simulink model "FOC_Motor_Control"  (R2020b)
settings: Solver=FixedStepAuto  StartTime=0.0  StopTime=10.0  FixedStep=Fixed_Step_Size  RelTol=1e-3
values from neighbouring files (symbols this model uses):
  atan_table = -1.5690511 -1.5690503 -1.5690495 -1.5690485 -1.5690477 -1.5690469 -1.569046 -1.5690452 -1.5690442 -1.5690434 -1.5690426 -1.5690417 -1.5690409 -1.5690399 -1.5690391 -1.5690383 -1.5690374 -1.5690365 -1.5690356 -1.5690348 -1.5690339 -1.569033 -1.5690322 -1.5690314 -1.5690304 -1.5690296 -1.5690287 -1.5690278 -1.5690269 -1.5690261 -1.5690252 -1.5690243 -1.5690234 -1.5690225 -1.5690217 -1.5690207 -1.569    [Motor_Control_Data.sldd]
  Cosine_table = 1.0 0.99999529 0.99999058 0.99998587 0.99998116 0.99996704 0.99995291 0.99993885 0.99992472 0.99990118 0.99987763 0.99985409 0.9998306 0.99979764 0.99976468 0.99973178 0.99969882 0.99965644 0.99961412 0.99957174 0.99952942 0.99947762 0.99942589 0.99937415 0.99932235 0.9992612 0.99920005 0.99913889 0.99907768 0.99900717 0.99893659 0.99886602 0.99879545 0.99871546 0.99863547 0.99855554 0.99847555 0.    [Motor_Control_Data.sldd]
  Dead_Com_Enable = 1.0    [Motor_Control_Data.sldd]
  Dead_Time = 2.5E-6    [Motor_Control_Data.sldd]
  Flux = 0.1125    [Motor_Control_Data.sldd]
  ID_Ki = 48.0    [Motor_Control_Data.sldd]
  ID_Kp = 0.84    [Motor_Control_Data.sldd]
  IQ_Ki = 48.0    [Motor_Control_Data.sldd]
  IQ_Kp = 1.869    [Motor_Control_Data.sldd]
  Ld = 0.00014    [Motor_Control_Data.sldd]
  Lq = 0.0003115    [Motor_Control_Data.sldd]
  Pole_Pairs = 4.0    [Motor_Control_Data.sldd]
  PWM_Frequency = 10000.0    [Motor_Control_Data.sldd]
  Sine_table = 0.0 0.0015339879 0.0030679768 0.0046019657 0.0061359555 0.0076698866 0.0092038177 0.010737749 0.012271681 0.013805497 0.015339312 0.016873131 0.018406944 0.019940587 0.021474229 0.023007872 0.024541514 0.026074925 0.027608337 0.029141748 0.03067516 0.032208283 0.033741407 0.035274528 0.036807653 0.038340431 0.039873205 0.04140598 0.042938754 0.04447113 0.046003502 0.047535874 0.049068246 0.0506001    [Motor_Control_Data.sldd]
  Speed_Ki = 10.809    [Motor_Control_Data.sldd]
  Speed_Kp = 0.08    [Motor_Control_Data.sldd]
  Speed_PI_OutputMax = 700.0    [Motor_Control_Data.sldd]
  Speed_PI_OutputMin = -700.0    [Motor_Control_Data.sldd]
  SpeedFilter_Fn = 0.2    [Motor_Control_Data.sldd]
  TorqueMode = 0.0    [Motor_Control_Data.sldd]
undefined symbols (not defined in the file or in its folder): DiscIntNeverNeededParam, inverter, LADRC_b0, LADRC_Omega_c, SVPWM
libraries: simulink x6
(part 2 of 2)

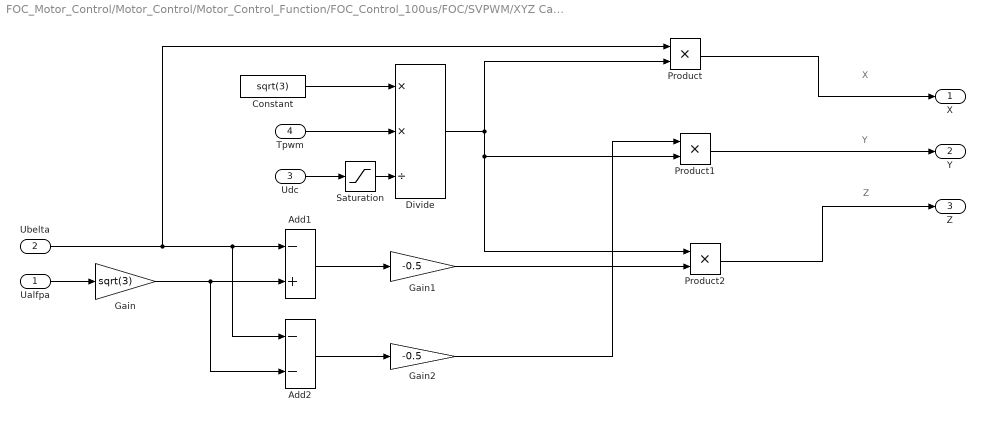
== system FOC_Motor_Control/Motor_Control/Motor_Control_Function/FOC_Control_100us/FOC/SVPWM/XYZ Caculate ==
  note: X
  note: Y
  note: Z
  Ualfpa : Inport
  Ubelta : Inport  Port=2
  Udc : Inport  Port=3
  Tpwm : Inport  Port=4
  Add1 : Sum  Inputs=-+
  Add2 : Sum  Inputs=--
  Constant : Constant  Value=sqrt(3)  OutDataTypeStr=single
  Divide : Product  Inputs=**/
  Gain : Gain  Gain=sqrt(3)
  Gain1 : Gain  Gain=-0.5
  Gain2 : Gain  Gain=-0.5
  Product : Product
  Product1 : Product
  Product2 : Product
  Saturation : Saturate  UpperLimit=1200  LowerLimit=0.0001
  X : Outport
  Y : Outport  Port=2
  Z : Outport  Port=3
  wires:
  Gain2/1 -> Product1/1
  Add2/1 -> Gain2/1
  Add1/1 -> Gain1/1
  Gain/1 -> Add2/2, Add1/2
  Ualfpa/1 -> Gain/1
  Ubelta/1 -> Add2/1, Add1/1, Product/1
  Gain1/1 -> Product2/2
  Product2/1 -> Z/1
  Divide/1 -> Product1/2, Product2/1, Product/2
  Product1/1 -> Y/1
  Product/1 -> X/1
  Udc/1 -> Saturation/1
  Tpwm/1 -> Divide/2
  Constant/1 -> Divide/1
  Saturation/1 -> Divide/3

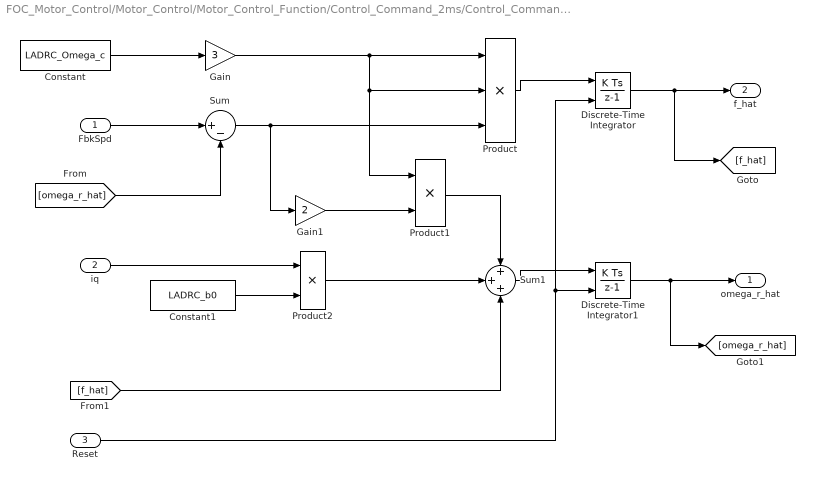
== system FOC_Motor_Control/Motor_Control/Motor_Control_Function/Control_Command_2ms/Control_Command_2ms/Speed_PI/SpeedLoop/LESO ==
  FbkSpd : Inport  OutDataTypeStr=single  PortDimensions=1
  iq : Inport  Port=2  OutDataTypeStr=single  PortDimensions=1
  Reset : Inport  Port=3
  Constant : Constant  Value=LADRC_Omega_c  OutDataTypeStr=single
  Constant1 : Constant  Value=LADRC_b0  OutDataTypeStr=single  SampleTime=-1
  Discrete-Time Integrator : DiscreteIntegrator  ExternalReset=level  SampleTime=-1  OutDataTypeStr=single  UpperSaturationLimit=6e4  LowerSaturationLimit=-6e4  ICPrevOutput=DiscIntNeverNeededParam  ICPrevScaledInput=DiscIntNeverNeededParam
  Discrete-Time Integrator1 : DiscreteIntegrator  ExternalReset=level  SampleTime=-1  OutDataTypeStr=single  LimitOutput=on  UpperSaturationLimit=2000  LowerSaturationLimit=-2000  ICPrevOutput=DiscIntNeverNeededParam  ICPrevScaledInput=DiscIntNeverNeededParam
  Gain : Gain  Gain=3  OutDataTypeStr=single
  Gain1 : Gain  Gain=2  OutDataTypeStr=single
  Product : Product  Inputs=3  OutDataTypeStr=single
  Product1 : Product  OutDataTypeStr=single
  Product2 : Product  OutDataTypeStr=single
  Sum : Sum  Inputs=|+-  OutDataTypeStr=single
  Sum1 : Sum  Inputs=+++  OutDataTypeStr=single
  omega_r_hat : Outport  OutDataTypeStr=single
  f_hat : Outport  Port=2  OutDataTypeStr=single
  wires:
  Sum/1 -> Gain1/1, Product/3
  Product/1 -> Discrete-Time Integrator/1
  Discrete-Time Integrator/1 -> [f_hat], f_hat/1
  [f_hat] -> Sum1/3
  Sum1/1 -> Discrete-Time Integrator1/1
  Discrete-Time Integrator1/1 -> omega_r_hat/1, [omega_r_hat]
  Product1/1 -> Sum1/1
  FbkSpd/1 -> Sum/1
  [omega_r_hat] -> Sum/2
  Constant/1 -> Gain/1
  Gain1/1 -> Product1/2
  Gain/1 -> Product1/1, Product/2, Product/1
  iq/1 -> Product2/1
  Constant1/1 -> Product2/2
  Product2/1 -> Sum1/2
  Reset/1 -> Discrete-Time Integrator/2, Discrete-Time Integrator1/2

== system FOC_Motor_Control/Motor_Control/Motor_Control_Function/Control_Command_2ms/Control_Command_2ms/Speed_PI/Speed_PI/Speed_Control ==
  Err : Inport
  Reset : Inport  Port=2
  Add : Sum
  Cons : Constant  Value=0  OutDataTypeStr=single
  Discrete-Time Integrator : DiscreteIntegrator  ExternalReset=level  SampleTime=-1  ICPrevOutput=DiscIntNeverNeededParam  ICPrevScaledInput=DiscIntNeverNeededParam
  Ki : Constant  Value=Speed_Ki  OutDataTypeStr=single
  Kp : Constant  Value=Speed_Kp  OutDataTypeStr=single
  Product : Product
  Product1 : Product
  Relational Operator1 : RelationalOperator  Operator===  OutDataTypeStr=boolean  RndMeth=Simplest
  Saturation : Saturate  UpperLimit=Speed_PI_OutputMax  LowerLimit=Speed_PI_OutputMin
  Scope : Scope
  Switch : Switch  Criteria=u2 > Threshold
  Unit Delay3 : UnitDelay  SampleTime=-1  HasFrameUpgradeWarning=on
  PI_Out : Outport
  wires:
  Kp/1 -> Product/1
  Err/1 -> Switch/1, Product/2
  Switch/1 -> Product1/2
  Product1/1 -> Discrete-Time Integrator/1
  Product/1 -> Add/1
  Add/1 -> Relational Operator1/1, Saturation/1
  Saturation/1 -> Relational Operator1/2, PI_Out/1
  Discrete-Time Integrator/1 -> Add/2, Scope/1
  Relational Operator1/1 -> Unit Delay3/1
  Ki/1 -> Product1/1
  Unit Delay3/1 -> Switch/2
  Cons/1 -> Switch/3
  Reset/1 -> Discrete-Time Integrator/2

== system FOC_Motor_Control/Motor_Control/Motor_Control_Function/FOC_Control_100us/FOC/DT_Compensation/DT_Compensation/IsTheta_Cal ==
  Id : Inport
  Iq : Inport  Port=2
  d_theta : Inport  Port=3
  Add1 : Sum
  Angle_calibration : Subsystem
      settings: RTWSystemCode=Nonreusable function  RTWFcnNameOpts=Use subsystem name
  LPF : Subsystem
  LPF1 : Subsystem
  Scope2 : Scope  NumInputPorts=2
  Scope3 : Scope  NumInputPorts=2
  atan : Subsystem
  IsTheta : Outport
  wires:
  d_theta/1 -> Add1/2
  Angle_calibration/1(Angle_output) -> IsTheta/1
  Iq/1 -> LPF/1(u), Scope2/1
  Id/1 -> LPF1/1(u), Scope3/1
  LPF1/1(y) -> [B_Id], Scope3/2
  LPF/1(y) -> Scope2/2, [A_Iq]
  Add1/1 -> Angle_calibration/1(Angle_input)  "Itheta2"
  [A_Iq] -> atan/1(Id)
  [B_Id] -> atan/2(Iq)
  atan/1(Out1) -> Add1/1

== system FOC_Motor_Control/Motor_Control/Motor_Control_Function/FOC_Control_100us/FOC/DT_Compensation/DT_Compensation/Subsystem ==
  Err_Voltage : Inport
  Istheta : Inport  Port=2
  If1 : If  IfExpression=(u1 >5.75958)|(u1<=0.523598)  ElseIfExpressions=(u1 >0.523598)&(u1<=1.570796),(u1 >1.570796)&(u1<=2.617993),(u1 >2.617993)&(u1<=3.665191),(u1 >3.665191)&(u1<=4.7123889),(u1 >4.7123889)&(u1<=5.75958)  ShowElse=off
  Merge : Merge  Inputs=6
  Subsystem : Subsystem
  Subsystem1 : Subsystem
  Subsystem2 : Subsystem
  Subsystem3 : Subsystem
  Subsystem4 : Subsystem
  Subsystem5 : Subsystem
  Uabcc : Outport
  wires:
  Istheta/1 -> If1/1
  If1/1 -> Subsystem/Action
  If1/2 -> Subsystem1/Action
  If1/3 -> Subsystem2/Action
  If1/4 -> Subsystem3/Action
  If1/5 -> Subsystem4/Action
  If1/6 -> Subsystem5/Action
  Err_Voltage/1 -> Subsystem5/1(Voltage), Subsystem3/1(Voltage), Subsystem2/1(Voltage), Subsystem/1(Voltage), Subsystem1/1(Voltage), Subsystem4/1(Voltage)
  Merge/1 -> Uabcc/1
  Subsystem/1(Out1) -> Merge/1
  Subsystem1/1(Out1) -> Merge/2
  Subsystem2/1(Out1) -> Merge/3
  Subsystem3/1(Out1) -> Merge/4
  Subsystem4/1(Out1) -> Merge/5
  Subsystem5/1(Out1) -> Merge/6

== system FOC_Motor_Control/Motor_Control/Motor_Control_Function/FOC_Control_100us/FOC/DT_Compensation/DT_Compensation/Uabc_alphabeta ==
  Uabc : Inport
  Fcn : Fcn  Expr=(2/3)*(u(1)-0.5*u(2)-0.5*u(3))
  Fcn1 : Fcn  Expr=sqrt(1/3)*(u(2)-u(3))
  Ualpha : Outport
  Ubeta : Outport  Port=2
  wires:
  Fcn/1 -> Ualpha/1
  Fcn1/1 -> Ubeta/1
  Uabc/1 -> Fcn1/1, Fcn/1

== system FOC_Motor_Control/Motor_Control/Motor_Control_Function/FOC_Control_100us/FOC/D_Current_PI/ID_Control/Normal ==
  Bus_voltage : Inport
  Gain : Gain  Gain=1/sqrt(3)
  Gain1 : Gain  Gain=-1/sqrt(3)
  Out1 : Outport
  Out2 : Outport  Port=2
  wires:
  Bus_voltage/1 -> Gain1/1, Gain/1
  Gain/1 -> Out1/1
  Gain1/1 -> Out2/1

== system FOC_Motor_Control/Motor_Control/Motor_Control_Function/FOC_Control_100us/FOC/Q_Current_PI/IQ_Control/Normal ==
  Bus_voltage : Inport
  Gain : Gain  Gain=1/sqrt(3)
  Gain1 : Gain  Gain=-1/sqrt(3)
  Out1 : Outport
  Out2 : Outport  Port=2
  wires:
  Bus_voltage/1 -> Gain1/1, Gain/1
  Gain/1 -> Out1/1
  Gain1/1 -> Out2/1

== system FOC_Motor_Control/Motor_Control/Motor_Control_Function/FOC_Control_100us/FOC/DT_Compensation/DT_Compensation/IsTheta_Cal/Angle_calibration ==
  Angle_input : Inport
  If Action Subsystem1 : Subsystem  TreatAsAtomicUnit=on
  If Action Subsystem2 : Subsystem  TreatAsAtomicUnit=on
  If1 : If  IfExpression=u1 > 6.283185307
  Merge1 : Merge
  Angle_output : Outport
  wires:
  Merge1/1 -> Angle_output/1
  If1/1 -> If Action Subsystem2/Action
  If1/2 -> If Action Subsystem1/Action
  If Action Subsystem2/1(Out1) -> Merge1/1
  Angle_input/1 -> If Action Subsystem1/1(Angle_input), If Action Subsystem2/1(In1), If1/1
  If Action Subsystem1/1(Out1) -> Merge1/2

== system FOC_Motor_Control/Motor_Control/Motor_Control_Function/FOC_Control_100us/FOC/DT_Compensation/DT_Compensation/IsTheta_Cal/LPF ==
  u : Inport
  Add : Sum  Inputs=+-
  Add1 : Sum
  Constant1 : Constant  Value=0.005  OutDataTypeStr=single
  Divide1 : Product  Inputs=**
  Unit Delay : UnitDelay  SampleTime=-1  HasFrameUpgradeWarning=on
  y : Outport
  wires:
  Constant1/1 -> Divide1/1
  u/1 -> Add/1
  Add/1 -> Divide1/2
  Divide1/1 -> Add1/1
  Unit Delay/1 -> Add/2, Add1/2
  Add1/1 -> Unit Delay/1, y/1

== system FOC_Motor_Control/Motor_Control/Motor_Control_Function/FOC_Control_100us/FOC/DT_Compensation/DT_Compensation/IsTheta_Cal/LPF1 ==
  u : Inport
  Add : Sum  Inputs=+-
  Add1 : Sum
  Constant1 : Constant  Value=0.005  OutDataTypeStr=single
  Divide1 : Product  Inputs=**
  Unit Delay : UnitDelay  SampleTime=-1  HasFrameUpgradeWarning=on
  y : Outport
  wires:
  Constant1/1 -> Divide1/1
  u/1 -> Add/1
  Add/1 -> Divide1/2
  Divide1/1 -> Add1/1
  Unit Delay/1 -> Add/2, Add1/2
  Add1/1 -> Unit Delay/1, y/1

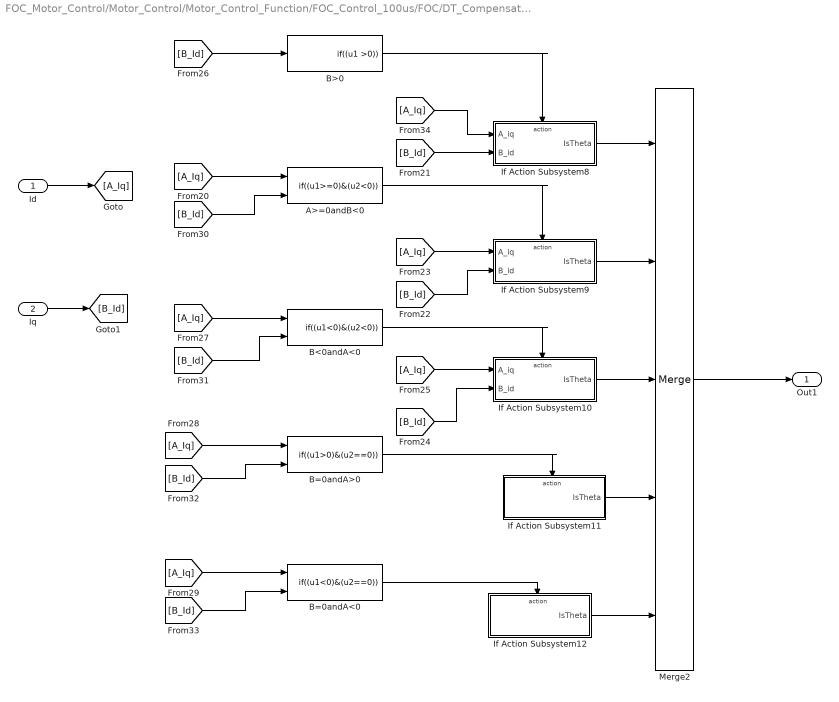
== system FOC_Motor_Control/Motor_Control/Motor_Control_Function/FOC_Control_100us/FOC/DT_Compensation/DT_Compensation/IsTheta_Cal/atan ==
  Id : Inport
  Iq : Inport  Port=2
  A>=0andB<0 : If  NumInputs=2  IfExpression=(u1>=0)&(u2<0)  ShowElse=off
  B<0andA<0 : If  NumInputs=2  IfExpression=(u1<0)&(u2<0)  ShowElse=off
  B=0andA<0 : If  NumInputs=2  IfExpression=(u1<0)&(u2==0)  ShowElse=off
  B=0andA>0 : If  NumInputs=2  IfExpression=(u1>0)&(u2==0)  ShowElse=off
  B>0 : If  IfExpression=(u1 >0)  ShowElse=off
  If Action Subsystem10 : Subsystem  TreatAsAtomicUnit=on
  If Action Subsystem11 : Subsystem  TreatAsAtomicUnit=on
  If Action Subsystem12 : Subsystem  TreatAsAtomicUnit=on
  If Action Subsystem8 : Subsystem  TreatAsAtomicUnit=on
  If Action Subsystem9 : Subsystem  TreatAsAtomicUnit=on
  Merge2 : Merge  Inputs=5
  Out1 : Outport
  wires:
  B<0andA<0/1 -> If Action Subsystem10/Action
  [A_Iq] -> If Action Subsystem10/1(A_iq)
  B=0andA<0/1 -> If Action Subsystem12/Action
  B=0andA>0/1 -> If Action Subsystem11/Action
  [A_Iq] -> If Action Subsystem8/1(A_iq)
  [B_Id] -> B>0/1
  A>=0andB<0/1 -> If Action Subsystem9/Action
  If Action Subsystem11/1(IsTheta) -> Merge2/4
  If Action Subsystem9/1(IsTheta) -> Merge2/2
  [B_Id] -> If Action Subsystem9/2(B_id)
  B>0/1 -> If Action Subsystem8/Action
  [A_Iq] -> If Action Subsystem9/1(A_iq)
  If Action Subsystem8/1(IsTheta) -> Merge2/1
  [B_Id] -> B<0andA<0/2
  [A_Iq] -> A>=0andB<0/1
  [B_Id] -> B=0andA<0/2
  [B_Id] -> A>=0andB<0/2
  [A_Iq] -> B=0andA<0/1
  [A_Iq] -> B=0andA>0/1
  [A_Iq] -> B<0andA<0/1
  [B_Id] -> B=0andA>0/2
  If Action Subsystem12/1(IsTheta) -> Merge2/5
  If Action Subsystem10/1(IsTheta) -> Merge2/3
  Merge2/1 -> Out1/1
  [B_Id] -> If Action Subsystem8/2(B_id)
  [B_Id] -> If Action Subsystem10/2(B_id)
  Id/1 -> [A_Iq]
  Iq/1 -> [B_Id]

== system FOC_Motor_Control/Motor_Control/Motor_Control_Function/FOC_Control_100us/FOC/DT_Compensation/DT_Compensation/Subsystem/Subsystem ==
  Voltage : Inport
  Action Port : ActionPort  ActionPortLabel=if((u1 >5.75958)|(u1<=0.523598))
  Gain : Gain
  Gain1 : Gain  Gain=-1
  Gain2 : Gain  Gain=-1
  Mux1 : Mux  Inputs=3
  Out1 : Outport
  wires:
  Gain/1 -> Mux1/1
  Gain1/1 -> Mux1/2
  Voltage/1 -> Gain2/1, Gain1/1, Gain/1
  Gain2/1 -> Mux1/3
  Mux1/1 -> Out1/1

== system FOC_Motor_Control/Motor_Control/Motor_Control_Function/FOC_Control_100us/FOC/DT_Compensation/DT_Compensation/Subsystem/Subsystem1 ==
  Voltage : Inport
  Action Port : ActionPort  ActionPortLabel=elseif((u1 >0.523598)&(u1<=1.570796))
  Gain : Gain
  Gain1 : Gain
  Gain2 : Gain  Gain=-1
  Mux1 : Mux  Inputs=3
  Out1 : Outport
  wires:
  Mux1/1 -> Out1/1
  Voltage/1 -> Gain2/1, Gain1/1, Gain/1
  Gain/1 -> Mux1/1
  Gain1/1 -> Mux1/2
  Gain2/1 -> Mux1/3

== system FOC_Motor_Control/Motor_Control/Motor_Control_Function/FOC_Control_100us/FOC/DT_Compensation/DT_Compensation/Subsystem/Subsystem2 ==
  Voltage : Inport
  Action Port : ActionPort  ActionPortLabel=elseif((u1 >1.570796)&(u1<=2.617993))
  Gain : Gain  Gain=-1
  Gain1 : Gain
  Gain2 : Gain  Gain=-1
  Mux1 : Mux  Inputs=3
  Out1 : Outport
  wires:
  Mux1/1 -> Out1/1
  Voltage/1 -> Gain2/1, Gain1/1, Gain/1
  Gain/1 -> Mux1/1
  Gain1/1 -> Mux1/2
  Gain2/1 -> Mux1/3

== system FOC_Motor_Control/Motor_Control/Motor_Control_Function/FOC_Control_100us/FOC/DT_Compensation/DT_Compensation/Subsystem/Subsystem3 ==
  Voltage : Inport
  Action Port : ActionPort  ActionPortLabel=elseif((u1 >2.617993)&(u1<=3.665191))
  Gain : Gain  Gain=-1
  Gain1 : Gain
  Gain2 : Gain
  Mux1 : Mux  Inputs=3
  Out1 : Outport
  wires:
  Mux1/1 -> Out1/1
  Voltage/1 -> Gain2/1, Gain1/1, Gain/1
  Gain/1 -> Mux1/1
  Gain1/1 -> Mux1/2
  Gain2/1 -> Mux1/3

== system FOC_Motor_Control/Motor_Control/Motor_Control_Function/FOC_Control_100us/FOC/DT_Compensation/DT_Compensation/Subsystem/Subsystem4 ==
  Voltage : Inport
  Action Port : ActionPort  ActionPortLabel=elseif((u1 >3.665191)&(u1<=4.7123889))
  Gain : Gain  Gain=-1
  Gain1 : Gain  Gain=-1
  Gain2 : Gain
  Mux1 : Mux  Inputs=3
  Out1 : Outport
  wires:
  Mux1/1 -> Out1/1
  Voltage/1 -> Gain2/1, Gain1/1, Gain/1
  Gain/1 -> Mux1/1
  Gain1/1 -> Mux1/2
  Gain2/1 -> Mux1/3

== system FOC_Motor_Control/Motor_Control/Motor_Control_Function/FOC_Control_100us/FOC/DT_Compensation/DT_Compensation/Subsystem/Subsystem5 ==
  Voltage : Inport
  Action Port : ActionPort  ActionPortLabel=elseif((u1 >4.7123889)&(u1<=5.75958))
  Gain : Gain
  Gain1 : Gain  Gain=-1
  Gain2 : Gain
  Mux1 : Mux  Inputs=3
  Out1 : Outport
  wires:
  Mux1/1 -> Out1/1
  Voltage/1 -> Gain2/1, Gain1/1, Gain/1
  Gain/1 -> Mux1/1
  Gain1/1 -> Mux1/2
  Gain2/1 -> Mux1/3

== system FOC_Motor_Control/Motor_Control/Motor_Control_Function/FOC_Control_100us/FOC/DT_Compensation/DT_Compensation/IsTheta_Cal/Angle_calibration/If Action Subsystem1 ==
  Angle_input : Inport
  Action Port : ActionPort  ActionPortLabel=else
  Out1 : Outport
  wires:
  Angle_input/1 -> Out1/1

== system FOC_Motor_Control/Motor_Control/Motor_Control_Function/FOC_Control_100us/FOC/DT_Compensation/DT_Compensation/IsTheta_Cal/Angle_calibration/If Action Subsystem2 ==
  In1 : Inport
  Action Port : ActionPort  ActionPortLabel=if(u1 > 6.283185307)
  2pi : Constant  Value=2*pi  OutDataTypeStr=single
  Subtract1 : Sum  Inputs=+-
  Out1 : Outport
  wires:
  In1/1 -> Subtract1/1
  Subtract1/1 -> Out1/1
  2pi/1 -> Subtract1/2

== system FOC_Motor_Control/Motor_Control/Motor_Control_Function/FOC_Control_100us/FOC/DT_Compensation/DT_Compensation/IsTheta_Cal/atan/If Action Subsystem10 ==
  A_iq : Inport
  B_id : Inport  Port=2
  Action Port : ActionPort  ActionPortLabel=if((u1<0)&(u2<0))
  1-D Lookup Table4 : Lookup_n-D  NumberOfTableDimensions=1  LookupTableObject=''  BreakpointsForDimension1=single(linspace(-573,573,length(atan_table)));  BreakpointsForDimension1FirstPoint=10  BreakpointsForDimension2FirstPoint=10  BreakpointsForDimension1Spacing=12  BreakpointsForDimension2Spacing=12  IndexSearchMethod=Evenly spaced points  Table=atan_table  InterpMethod=Flat  DiagnosticForOutOfRangeInput=Error  InternalRulePriority=Speed  RndMeth=Simplest  InputSameDT=on
  Add : Sum  Inputs=+-
  Constant : Constant  Value=pi  OutDataTypeStr=single
  Divide : Product  Inputs=*/
  Saturation : Saturate  UpperLimit=572  LowerLimit=-572
  Scope : Scope
  IsTheta : Outport
  wires:
  Add/1 -> IsTheta/1
  Saturation/1 -> Scope/1, 1-D Lookup Table4/1
  A_iq/1 -> Divide/1
  Constant/1 -> Add/2
  Divide/1 -> Saturation/1
  B_id/1 -> Divide/2
  1-D Lookup Table4/1 -> Add/1

== system FOC_Motor_Control/Motor_Control/Motor_Control_Function/FOC_Control_100us/FOC/DT_Compensation/DT_Compensation/IsTheta_Cal/atan/If Action Subsystem11 ==
  Action Port : ActionPort  ActionPortLabel=if((u1>0)&(u2==0))
  Constant : Constant  Value=pi/2  OutDataTypeStr=single
  IsTheta : Outport
  wires:
  Constant/1 -> IsTheta/1

== system FOC_Motor_Control/Motor_Control/Motor_Control_Function/FOC_Control_100us/FOC/DT_Compensation/DT_Compensation/IsTheta_Cal/atan/If Action Subsystem12 ==
  Action Port : ActionPort  ActionPortLabel=if((u1<0)&(u2==0))
  Constant : Constant  Value=-pi/2  OutDataTypeStr=single
  IsTheta : Outport
  wires:
  Constant/1 -> IsTheta/1

== system FOC_Motor_Control/Motor_Control/Motor_Control_Function/FOC_Control_100us/FOC/DT_Compensation/DT_Compensation/IsTheta_Cal/atan/If Action Subsystem8 ==
  A_iq : Inport
  B_id : Inport  Port=2
  Action Port : ActionPort  ActionPortLabel=if((u1 >0))
  1-D Lookup Table4 : Lookup_n-D  NumberOfTableDimensions=1  LookupTableObject=''  BreakpointsForDimension1=single(linspace(-573,573,length(atan_table)));  BreakpointsForDimension1FirstPoint=10  BreakpointsForDimension2FirstPoint=10  BreakpointsForDimension1Spacing=12  BreakpointsForDimension2Spacing=12  IndexSearchMethod=Evenly spaced points  Table=atan_table  InterpMethod=Flat  DiagnosticForOutOfRangeInput=Error  InternalRulePriority=Speed  RndMeth=Simplest  InputSameDT=on
  Divide : Product  Inputs=*/
  Saturation : Saturate  UpperLimit=572  LowerLimit=-572
  Scope : Scope  NumInputPorts=2
  IsTheta : Outport
  wires:
  Divide/1 -> Saturation/1
  A_iq/1 -> Divide/1
  B_id/1 -> Divide/2
  Saturation/1 -> Scope/1, 1-D Lookup Table4/1
  1-D Lookup Table4/1 -> Scope/2, IsTheta/1

== system FOC_Motor_Control/Motor_Control/Motor_Control_Function/FOC_Control_100us/FOC/DT_Compensation/DT_Compensation/IsTheta_Cal/atan/If Action Subsystem9 ==
  A_iq : Inport
  B_id : Inport  Port=2
  Action Port : ActionPort  ActionPortLabel=if((u1>=0)&(u2<0))
  1-D Lookup Table4 : Lookup_n-D  NumberOfTableDimensions=1  LookupTableObject=''  BreakpointsForDimension1=single(linspace(-573,573,length(atan_table)));  BreakpointsForDimension1FirstPoint=10  BreakpointsForDimension2FirstPoint=10  BreakpointsForDimension1Spacing=12  BreakpointsForDimension2Spacing=12  IndexSearchMethod=Evenly spaced points  Table=atan_table  InterpMethod=Flat  DiagnosticForOutOfRangeInput=Error  InternalRulePriority=Speed  RndMeth=Simplest  InputSameDT=on
  Add : Sum
  Constant : Constant  Value=pi  OutDataTypeStr=single
  Divide : Product  Inputs=*/
  Saturation : Saturate  UpperLimit=572  LowerLimit=-572
  Scope : Scope  NumInputPorts=3
  IsTheta : Outport
  wires:
  B_id/1 -> Divide/2
  A_iq/1 -> Divide/1
  Add/1 -> Scope/3, IsTheta/1
  Constant/1 -> Add/2
  Saturation/1 -> Scope/1, 1-D Lookup Table4/1
  Divide/1 -> Saturation/1
  1-D Lookup Table4/1 -> Scope/2, Add/1
